simulink model "Target_Control_System"  (R2021b)
settings: Solver=FixedStepDiscrete  StartTime=0.0  StopTime=5  RelTol=1e-3
PreLoadFcn:
  | RTWConfigurationCB('preloadfcn', bdroot);
PostLoadFcn:
  | load('configuration/data_struct.mat');
  | load('configuration/fluxMaps_propMotor.mat');
  | load('configuration/parameterInit_PROP.mat');
  | load('configuration/parameterInit_PUMP.mat');
  | load('configuration/parameterInit_PITCH.mat');
  | load('configuration/parameterInit_TILT.mat');
  | %load('configuration/base_workspace_signal_definition.mat');
  | %load('resolvedatastores_to_baseworkspace_for_faster_simulation.mat');
model workspace (MAT data in the model file):
  SIMULATION_OPTIONS : Simulink.Parameter (value not decoded)
  TARGET_CODE_GEN : Simulink.Parameter (value not decoded)
  TCS_SAMPLE_FREQ_HZ : Simulink.Parameter (value not decoded)
symbols that are objects in the model workspace (value not decoded): TARGET_CODE_GEN, TCS_SAMPLE_FREQ_HZ
undefined symbols (not defined in the file): A_DQ_REF_LPF_INIT__PITCH, A_DQ_REF_LPF_INIT__PROP, A_DQ_REF_LPF_INIT__PUMP, A_DQ_REF_LPF_INIT__TILT, A_OBSERVER_CONFIDENCE_INIT__PITCH, A_OBSERVER_CONFIDENCE_INIT__PROP, A_OBSERVER_CONFIDENCE_INIT__PUMP, A_OBSERVER_CONFIDENCE_INIT__TILT, ACTUATOR_MAX_ANGLE_TRIP__PITCH, ACTUATOR_MIN_ANGLE_TRIP__PITCH, ACTUATOR_POS_SENSOR_INV_DIRECTION__PITCH, ACTUATOR_POS_SENSOR_INV_DIRECTION__TILT, ACTUATOR_POS_SENSOR_OFFSET__PITCH, ACTUATOR_POS_SENSOR_OFFSET__TILT, ADC_scaler1_baseaddr_TILT, ADC_SCALER_FLOAT_TO_FIXPOINT_EXPANSION, ANGLE_ELEC_FROM_SENSOR_OFFSET_INIT__PITCH, ANGLE_ELEC_FROM_SENSOR_OFFSET_INIT__PROP, ANGLE_ELEC_FROM_SENSOR_OFFSET_INIT__PUMP, ANGLE_ELEC_FROM_SENSOR_OFFSET_INIT__TILT, AUTO_CLEAR_FAULTS_ENABLED__PITCH, AUTO_CLEAR_FAULTS_ENABLED__PROP, AUTO_CLEAR_FAULTS_ENABLED__PUMP, AUTO_CLEAR_FAULTS_ENABLED__TILT, AUTO_CLEAR_FAULTS_WAIT_TICKS__PITCH, AUTO_CLEAR_FAULTS_WAIT_TICKS__PROP, AUTO_CLEAR_FAULTS_WAIT_TICKS__PUMP, AUTO_CLEAR_FAULTS_WAIT_TICKS__TILT, AUTO_I_ZERO_IDLE_TICKS__PITCH, AUTO_I_ZERO_IDLE_TICKS__PROP, AUTO_I_ZERO_IDLE_TICKS__PUMP, AUTO_I_ZERO_IDLE_TICKS__TILT, AUTO_I_ZERO_OFFSET_IDC_THRESHOLD__PITCH, AUTO_I_ZERO_OFFSET_IDC_THRESHOLD__PROP, AUTO_I_ZERO_OFFSET_IDC_THRESHOLD__PUMP, AUTO_I_ZERO_OFFSET_IDC_THRESHOLD__TILT, AUTO_I_ZERO_OFFSET_IPH_THRESHOLD__PITCH, AUTO_I_ZERO_OFFSET_IPH_THRESHOLD__PROP, AUTO_I_ZERO_OFFSET_IPH_THRESHOLD__PUMP, AUTO_I_ZERO_OFFSET_IPH_THRESHOLD__TILT, AUTO_SENSORLESS_SWITCHOVER_DISABLE_OMEGA, AUTO_SENSORLESS_SWITCHOVER_ENABLE_OMEGA, AUTO_SENSORLESS_SWITCHOVER_MIN_CONFIDENCE, AUXILIARY_PROTECTION_UNIT_BASEADDR__TILT, blanking_max_error_omega_INIT_PITCH, blanking_max_error_omega_INIT_TILT, blanking_max_error_position_INIT_PITCH, blanking_max_error_position_INIT_TILT, BRUTE_START_I_Q_REF_RAMP_SPEED__PITCH, BRUTE_START_I_Q_REF_RAMP_SPEED__PROP, BRUTE_START_I_Q_REF_RAMP_SPEED__PUMP, BRUTE_START_I_Q_REF_RAMP_SPEED__TILT, CONTROL_LOOP_DT_INIT__PITCH, CONTROL_LOOP_DT_INIT__PROP, CONTROL_LOOP_DT_INIT__PUMP, CONTROL_LOOP_DT_INIT__TILT, CORRECTION_FILTER_SCALE__PITCH, CORRECTION_FILTER_SCALE__PROP, CORRECTION_FILTER_SCALE__PUMP, CORRECTION_FILTER_SCALE__TILT ... (+458)
libraries: simulink x178, Reusables_Lib x24
(part 36 of 47)

== system Target_Control_System/Target_Control_System/Simulation Controls/Simulation Data Store Initialization/setupPwm()/setPwmFrequencyApplication()_pitch/setPwmFrequency()_pitch/softwareIirFilterInitialize()1 ==
  fFreq3db : Inport
  fFreqSample : Inport  Port=2
  Constant : Constant  OutDataTypeStr=single  SampleTime=-1
  Constant1 : Constant  Value=0  OutDataTypeStr=single  SampleTime=-1
  Data Store Write : DataStoreWrite  DataStoreName=oPitch  DataStoreElements=oPitch.oMot_.oState_.oFilterDataForSpeedControlIqRef_.afConstantsA_.h0  IndexOptions=Index vector (dialog)  Indices=1  OutputSizes=1
  Data Store Write1 : DataStoreWrite  DataStoreName=oPitch  DataStoreElements=oPitch.oMot_.oState_.oFilterDataForSpeedControlIqRef_.afConstantsA_.h1  IndexOptions=Index vector (dialog)  Indices=1  OutputSizes=1
  Data Store Write10 : DataStoreWrite  DataStoreName=oPitch  DataStoreElements=oPitch.oMot_.oState_.oFilterDataForSpeedControlIqRef_.fFilterOutput_  IndexOptions=Index vector (dialog)  Indices=1  OutputSizes=1
  Data Store Write2 : DataStoreWrite  DataStoreName=oPitch  DataStoreElements=oPitch.oMot_.oState_.oFilterDataForSpeedControlIqRef_.afConstantsA_.h2  IndexOptions=Index vector (dialog)  Indices=1  OutputSizes=1
  Data Store Write3 : DataStoreWrite  DataStoreName=oPitch  DataStoreElements=oPitch.oMot_.oState_.oFilterDataForSpeedControlIqRef_.afConstantsB_.h2  IndexOptions=Index vector (dialog)  Indices=1  OutputSizes=1
  Data Store Write4 : DataStoreWrite  DataStoreName=oPitch  DataStoreElements=oPitch.oMot_.oState_.oFilterDataForSpeedControlIqRef_.afConstantsB_.h1  IndexOptions=Index vector (dialog)  Indices=1  OutputSizes=1
  Data Store Write5 : DataStoreWrite  DataStoreName=oPitch  DataStoreElements=oPitch.oMot_.oState_.oFilterDataForSpeedControlIqRef_.afConstantsB_.h0  IndexOptions=Index vector (dialog)  Indices=1  OutputSizes=1
  Data Store Write6 : DataStoreWrite  DataStoreName=oPitch  DataStoreElements=oPitch.oMot_.oState_.oFilterDataForSpeedControlIqRef_.afPreviousInputs_.h0  IndexOptions=Index vector (dialog)  Indices=1  OutputSizes=1
  Data Store Write7 : DataStoreWrite  DataStoreName=oPitch  DataStoreElements=oPitch.oMot_.oState_.oFilterDataForSpeedControlIqRef_.afPreviousInputs_.h1  IndexOptions=Index vector (dialog)  Indices=1  OutputSizes=1
  Data Store Write8 : DataStoreWrite  DataStoreName=oPitch  DataStoreElements=oPitch.oMot_.oState_.oFilterDataForSpeedControlIqRef_.afPreviousOutputs_.h0  IndexOptions=Index vector (dialog)  Indices=1  OutputSizes=1
  Data Store Write9 : DataStoreWrite  DataStoreName=oPitch  DataStoreElements=oPitch.oMot_.oState_.oFilterDataForSpeedControlIqRef_.afPreviousOutputs_.h1  IndexOptions=Index vector (dialog)  Indices=1  OutputSizes=1
  Data Type Conversion{1..5} (5 alike) : DataTypeConversion  OutDataTypeStr=single
  Demux : Demux  Outputs=6
  Divide : Product  Inputs=*/  OutDataTypeStr=single
  computeCoefficientsButter() : Subsystem
  fActualFrequencyHz : Outport
  wires:
  Data Type Conversion5/1 -> Data Store Write2/1
  Data Type Conversion4/1 -> Data Store Write1/1
  Data Type Conversion3/1 -> Data Store Write3/1
  Data Type Conversion2/1 -> Data Store Write4/1
  Data Type Conversion1/1 -> Data Store Write5/1
  fFreqSample/1 -> computeCoefficientsButter()/2(dSampleFrequencyHz)
  Constant1/1 -> Data Store Write6/1, Data Store Write7/1, Data Store Write9/1, Data Store Write10/1, Data Store Write8/1
  Demux/1 -> Data Type Conversion1/1
  Demux/2 -> Data Type Conversion2/1
  Constant/1 -> Divide/1
  Divide/1 -> Data Store Write/1
  Demux/4 -> Divide/2
  Demux/3 -> Data Type Conversion3/1
  Demux/5 -> Data Type Conversion4/1
  Demux/6 -> Data Type Conversion5/1
  computeCoefficientsButter()/1(dpOutArray) -> Demux/1
  fFreq3db/1 -> computeCoefficientsButter()/1(fCutoffFrequencyHz)
  computeCoefficientsButter()/2(fFreq3db) -> fActualFrequencyHz/1

== system Target_Control_System/Target_Control_System/Simulation Controls/Simulation Data Store Initialization/setupPwm()/setPwmFrequencyApplication()_pitch/setPwmFrequency()_pitch/updateObserver()_pitch ==
  oIsr_.oParam_.fControlLoopDt_ : Inport
  fObserverLoopFilterBandwidthHz_ : Inport  Port=2
  Constant : Constant  Value=15*2*pi  OutDataTypeStr=single
  Constant1 : Constant  Value=8*2*pi  OutDataTypeStr=single
  Constant2 : Constant  Value=2*pi  OutDataTypeStr=single
  Constant3 : Constant  Value=500  OutDataTypeStr=single
  Constant4 : Constant  Value=20  OutDataTypeStr=single
  Constant5 : Constant  Value=100*2*pi  OutDataTypeStr=single
  Constant6 : Constant  Value=4*2*pi  OutDataTypeStr=single
  Constant7 : Constant  Value=0.0625  OutDataTypeStr=single
  Data Store Write : DataStoreWrite  DataStoreName=oPitch  DataStoreElements=oPitch.oIsr_.oParam_.fALpf4hpfDcBlocking_  IndexOptions=Index vector (dialog)  Indices=1  OutputSizes=1
  Data Store Write1 : DataStoreWrite  DataStoreName=oPitch  DataStoreElements=oPitch.oIsr_.oParam_.fAFluxMagnitude_  IndexOptions=Index vector (dialog)  Indices=1  OutputSizes=1
  Data Store Write2 : DataStoreWrite  DataStoreName=oPitch  DataStoreElements=oPitch.oIsr_.oParam_.fALoopfilter2_  IndexOptions=Index vector (dialog)  Indices=1  OutputSizes=1
  Data Store Write3 : DataStoreWrite  DataStoreName=oPitch  DataStoreElements=oPitch.oMot_.oParam_.fObserverLoopFilterBandwidthHz_  IndexOptions=Index vector (dialog)  Indices=1  OutputSizes=1
  Data Store Write4 : DataStoreWrite  DataStoreName=oPitch  DataStoreElements=oPitch.oIsr_.oParam_.fAOmegaFilter2_  IndexOptions=Index vector (dialog)  Indices=1  OutputSizes=1
  Data Store Write5 : DataStoreWrite  DataStoreName=oPitch  DataStoreElements=oPitch.oMot_.oParam_.fAOmegaXfilter2_  IndexOptions=Index vector (dialog)  Indices=1  OutputSizes=1
  Data Store Write6 : DataStoreWrite  DataStoreName=oPitch  DataStoreElements=oPitch.oIsr_.oParam_.oPiDataPll2_.oParameter_.fKp_  IndexOptions=Index vector (dialog)  Indices=1  OutputSizes=1
  Divide{,1,3..4} (4 alike) : Product  Inputs=**
  Divide2 : Product  Inputs=***
  Divide5 : Product  Inputs=*/
  GreaterThan : RelationalOperator  Operator=<  OutDataTypeStr=boolean  RndMeth=Simplest
  Saturation{,1..4} (5 alike) : Saturate  UpperLimit=1.0  LowerLimit=1e-6
  Switch : Switch  Criteria=u2 > Threshold
  wires:
  Divide5/1 -> Data Store Write6/1
  Constant7/1 -> Divide5/1
  Saturation4/1 -> Data Store Write5/1
  oIsr_.oParam_.fControlLoopDt_/1 -> Divide/1, Divide1/1, Divide3/1, Divide2/2, Divide5/2, Divide4/1
  Divide4/1 -> Saturation4/1
  Constant6/1 -> Divide4/2
  Saturation3/1 -> Data Store Write4/1
  Divide3/1 -> Saturation3/1
  Constant5/1 -> Divide3/2
  Switch/1 -> Data Store Write3/1, Divide2/1
  Constant3/1 -> Switch/1
  GreaterThan/1 -> Switch/2
  Constant4/1 -> GreaterThan/2
  fObserverLoopFilterBandwidthHz_/1 -> Switch/3, GreaterThan/1
  Divide2/1 -> Saturation2/1
  Saturation2/1 -> Data Store Write2/1
  Constant2/1 -> Divide2/3
  Divide1/1 -> Saturation1/1
  Saturation1/1 -> Data Store Write1/1
  Constant1/1 -> Divide1/2
  Saturation/1 -> Data Store Write/1
  Divide/1 -> Saturation/1
  Constant/1 -> Divide/2

== system Target_Control_System/Target_Control_System/Simulation Controls/Simulation Data Store Initialization/setupPwm()/setPwmFrequencyApplication()_pitch/setPwmFrequency()_pitch/updateServoObserver()_pitch ==
  oIsr_.oParam_.fControlLoopDt_ : Inport  OutDataTypeStr=double
  fOmegaEDifferentiatorBandwidthHz_ : Inport  Port=2
  Constant : Constant  OutDataTypeStr=single
  Data Store Write : DataStoreWrite  DataStoreName=oPitch  DataStoreElements=oPitch.oMot_.oState_.oPosSensor_.fOmegaEDifferentiatorBandwidthHz_  IndexOptions=Index vector (dialog)  Indices=1  OutputSizes=1
  Divide : Product  Inputs=*/  OutDataTypeStr=single
  softwareIirFilterInitialize() : Subsystem  TreatAsAtomicUnit=on
  wires:
  fOmegaEDifferentiatorBandwidthHz_/1 -> softwareIirFilterInitialize()/1(fFreq3db)
  Divide/1 -> softwareIirFilterInitialize()/2(fFreqSample)
  oIsr_.oParam_.fControlLoopDt_/1 -> Divide/2
  softwareIirFilterInitialize()/1(fActualFrequencyHz) -> Data Store Write/1
  Constant/1 -> Divide/1

== system Target_Control_System/Target_Control_System/Simulation Controls/Simulation Data Store Initialization/updateServoObserver(&oTilt)/updateServoObserver()/softwareIirFilterInitialize()/computeCoefficientsButter() ==
  fCutoffFrequencyHz : Inport  OutDataTypeStr=single
  dSampleFrequencyHz : Inport  Port=2  OutDataTypeStr=single
  Add : Sum  Inputs=+++  OutDataTypeStr=double
  Add1 : Sum  Inputs=-+
  Add2 : Sum  Inputs=+-+  OutDataTypeStr=double
  Constant : Constant  Value=0.0008  OutDataTypeStr=single
  Constant1 : Constant  Value=0.45  OutDataTypeStr=single
  Constant{5,7,9..10} (4 alike) : Constant
  Constant2 : Constant  Value=pi  OutDataTypeStr=double
  Constant3 : Constant  OutDataTypeStr=double
  Constant4 : Constant  Value=sqrt(2)  OutDataTypeStr=double
  Constant6 : Constant  OutDataTypeStr=double
  Constant8 : Constant  Value=2
  Data Type Conversion : DataTypeConversion  OutDataTypeStr=double
  Divide : Product  Inputs=**  OutDataTypeStr=single
  Divide1 : Product  Inputs=**  OutDataTypeStr=single
  Divide{3,5..6,8,10..11} (6 alike) : Product  Inputs=**  OutDataTypeStr=double
  Divide2 : Product  Inputs=*/  OutDataTypeStr=double
  Divide4 : Product  Inputs=*/  OutDataTypeStr=double
  Divide7 : Product  Inputs=*/  OutDataTypeStr=double
  Divide9 : Product  Inputs=***  OutDataTypeStr=double
  Gain : Gain  Gain=2  OutDataTypeStr=double
  Gain1 : Gain  Gain=-1  OutDataTypeStr=double
  Gain2 : Gain  Gain=-1  OutDataTypeStr=double
  Gain3 : Gain  Gain=-1  OutDataTypeStr=double
  Mux : Mux  Inputs=6
  Saturation Dynamic : simulink/Discontinuities/Saturation Dynamic  OutMin=[]  OutMax=[]  OutDataTypeStr=Inherit: Same as second input  OutDataType=fixdt(1, 16)  OutScaling=2^-10  DoSatur=off
  Tan : Trigonometry  Operator=tan
  dpOutArray : Outport
  fFreq3db : Outport  Port=2
  wires:
  Data Type Conversion/1 -> Divide2/1
  Constant10/1 -> Mux/4
  [dA2] -> Gain3/1
  Gain3/1 -> Mux/6
  [dA1] -> Gain2/1
  Gain2/1 -> Mux/5
  [dB2] -> Mux/3
  [dB1] -> Mux/2
  [dB0] -> Mux/1
  Divide11/1 -> [dA2]
  Gain1/1 -> Divide11/2
  Add2/1 -> Gain1/1
  Constant9/1 -> Add2/3
  Divide10/1 -> Add2/2
  [kdQ] -> Divide10/2
  Constant7/1 -> Add1/1
  Divide8/1 -> Add1/2, Add2/1
  Divide9/1 -> [dA1]
  Constant8/1 -> Divide9/3
  Add1/1 -> Divide9/2
  [kdIta] -> Divide8/1, Divide8/2, Divide10/1
  Gain/1 -> [dB1]
  Divide7/1 -> [dB0], Gain/1, [dB2], Divide9/1, Divide11/1
  Add/1 -> Divide7/2
  Constant6/1 -> Divide7/1
  Constant5/1 -> Add/3
  Divide5/1 -> Add/2
  Divide6/1 -> Add/1
  [kdQ] -> Divide5/2
  [kdIta] -> Divide5/1, Divide6/1, Divide6/2
  Mux/1 -> dpOutArray/1
  Constant4/1 -> [kdQ]
  Divide4/1 -> [kdIta]
  Constant3/1 -> Divide4/1
  Tan/1 -> Divide4/2
  Divide3/1 -> Tan/1
  Constant2/1 -> Divide3/2
  Divide2/1 -> Divide3/1  "dFf"
  Constant/1 -> Divide/2
  Saturation Dynamic/1 -> fFreq3db/1, Data Type Conversion/1  "fCutoffFrequencyHz"
  Divide1/1 -> Saturation Dynamic/1
  dSampleFrequencyHz/1 -> Divide1/2, Divide2/2, Divide/1
  Constant1/1 -> Divide1/1
  Divide/1 -> Saturation Dynamic/3
  fCutoffFrequencyHz/1 -> Saturation Dynamic/2

== system Target_Control_System/Target_Control_System/Simulation Controls/Simulation Data Store Initialization/updateServoObserver()/updateServoObserver()_pitch/softwareIirFilterInitialize()/computeCoefficientsButter() ==
  fCutoffFrequencyHz : Inport  OutDataTypeStr=single
  dSampleFrequencyHz : Inport  Port=2  OutDataTypeStr=single
  Add : Sum  Inputs=+++  OutDataTypeStr=double
  Add1 : Sum  Inputs=-+
  Add2 : Sum  Inputs=+-+  OutDataTypeStr=double
  Constant : Constant  Value=0.0008  OutDataTypeStr=single  SampleTime=-1
  Constant1 : Constant  Value=0.45  OutDataTypeStr=single  SampleTime=-1
  Constant{5,7,9..10} (4 alike) : Constant  SampleTime=-1
  Constant2 : Constant  Value=pi  OutDataTypeStr=double  SampleTime=-1
  Constant3 : Constant  OutDataTypeStr=double  SampleTime=-1
  Constant4 : Constant  Value=sqrt(2)  OutDataTypeStr=double  SampleTime=-1
  Constant6 : Constant  OutDataTypeStr=double  SampleTime=-1
  Constant8 : Constant  Value=2  SampleTime=-1
  Data Type Conversion : DataTypeConversion  OutDataTypeStr=double
  Divide : Product  Inputs=**  OutDataTypeStr=single
  Divide1 : Product  Inputs=**  OutDataTypeStr=single
  Divide{3,5..6,8,10..11} (6 alike) : Product  Inputs=**  OutDataTypeStr=double
  Divide2 : Product  Inputs=*/  OutDataTypeStr=double
  Divide4 : Product  Inputs=*/  OutDataTypeStr=double
  Divide7 : Product  Inputs=*/  OutDataTypeStr=double
  Divide9 : Product  Inputs=***  OutDataTypeStr=double
  Gain : Gain  Gain=2  OutDataTypeStr=double
  Gain1 : Gain  Gain=-1  OutDataTypeStr=double
  Gain2 : Gain  Gain=-1  OutDataTypeStr=double
  Gain3 : Gain  Gain=-1  OutDataTypeStr=double
  Mux : Mux  Inputs=6
  Saturation Dynamic : simulink/Discontinuities/Saturation Dynamic  OutMin=[]  OutMax=[]  OutDataTypeStr=Inherit: Same as second input  OutDataType=fixdt(1, 16)  OutScaling=2^-10  DoSatur=off
  Tan : Trigonometry  Operator=tan
  dpOutArray : Outport
  fFreq3db : Outport  Port=2
  wires:
  Data Type Conversion/1 -> Divide2/1
  Constant10/1 -> Mux/4
  [dA2] -> Gain3/1
  Gain3/1 -> Mux/6
  [dA1] -> Gain2/1
  Gain2/1 -> Mux/5
  [dB2] -> Mux/3
  [dB1] -> Mux/2
  [dB0] -> Mux/1
  Divide11/1 -> [dA2]
  Gain1/1 -> Divide11/2
  Add2/1 -> Gain1/1
  Constant9/1 -> Add2/3
  Divide10/1 -> Add2/2
  [kdQ] -> Divide10/2
  Constant7/1 -> Add1/1
  Divide8/1 -> Add1/2, Add2/1
  Divide9/1 -> [dA1]
  Constant8/1 -> Divide9/3
  Add1/1 -> Divide9/2
  [kdIta] -> Divide8/1, Divide8/2, Divide10/1
  Gain/1 -> [dB1]
  Divide7/1 -> [dB0], Gain/1, [dB2], Divide9/1, Divide11/1
  Add/1 -> Divide7/2
  Constant6/1 -> Divide7/1
  Constant5/1 -> Add/3
  Divide5/1 -> Add/2
  Divide6/1 -> Add/1
  [kdQ] -> Divide5/2
  [kdIta] -> Divide5/1, Divide6/1, Divide6/2
  Mux/1 -> dpOutArray/1
  Constant4/1 -> [kdQ]
  Divide4/1 -> [kdIta]
  Constant3/1 -> Divide4/1
  Tan/1 -> Divide4/2
  Divide3/1 -> Tan/1
  Constant2/1 -> Divide3/2
  Divide2/1 -> Divide3/1  "dFf"
  Constant/1 -> Divide/2
  Saturation Dynamic/1 -> fFreq3db/1, Data Type Conversion/1  "fCutoffFrequencyHz"
  Divide1/1 -> Saturation Dynamic/1
  dSampleFrequencyHz/1 -> Divide1/2, Divide2/2, Divide/1
  Constant1/1 -> Divide1/1
  Divide/1 -> Saturation Dynamic/3
  fCutoffFrequencyHz/1 -> Saturation Dynamic/2

== system Target_Control_System/Target_Control_System/MainLoop/pitchMotor_mainLoop/Decimation gate for 10 Hz Pitch/Function-Call Subsystem/Dynamic_current_limiting_pitch/Enabled Subsystem/Enabled Subsystem ==
  Enable : EnablePort
  Constant2 : Constant  Value=0  OutDataTypeStr=uint32  SampleTime=-1
  Constant4 : Constant  Value=0  OutDataTypeStr=uint32  SampleTime=-1
  Data Store Write5 : DataStoreWrite  DataStoreName=oPitch  DataStoreElements=oPitch.oMot_.oOut_.uiEnableGateDrive_  IndexOptions=Index vector (dialog)  Indices=1  OutputSizes=1
  Data Store Write6 : DataStoreWrite  DataStoreName=oPitch  DataStoreElements=oPitch.oMot_.oOut_.uiCurrentControllerActive_  IndexOptions=Index vector (dialog)  Indices=1  OutputSizes=1
  wires:
  Constant2/1 -> Data Store Write5/1
  Constant4/1 -> Data Store Write6/1

== system Target_Control_System/Target_Control_System/MainLoop/pitchMotor_mainLoop/Decimation gate for 200 Hz Pitch/Function-Call Subsystem/Forced current injection for broken input sensors/Enabled Subsystem/Pure_0rpm_holding_mode ==
  Enable : EnablePort
  Constant : Constant  Value=0  OutDataTypeStr=single  SampleTime=-1
  Data Store Write : DataStoreWrite  DataStoreName=oPitch  DataStoreElements=oPitch.oMot_.oState_.oRampDataOmegaERef_.fSetpoint_  IndexOptions=Index vector (dialog)  Indices=1  OutputSizes=1
  Data Store Write1 : DataStoreWrite  DataStoreName=oPitch  DataStoreElements=oPitch.oMot_.oState_.oRampDataOmegaERef_.fRampOut_  IndexOptions=Index vector (dialog)  Indices=1  OutputSizes=1
  wires:
  Constant/1 -> Data Store Write/1, Data Store Write1/1

== system Target_Control_System/Target_Control_System/MainLoop/pitchMotor_mainLoop/Decimation gate for 200 Hz Pitch/Function-Call Subsystem/Forced current injection for broken input sensors/Enabled Subsystem/Rudimentary_forced_angle_position_control ==
  note: // (fErrorReduction_ assumed to be gte 0)
  note: // Limit maximum speed
  note: // Reduce top speed 33-fold
  Enable : EnablePort
  Abs1 : Abs
  Add2 : Sum  Inputs=+-
  Add3 : Sum  Inputs=+-
  Data Store Read : DataStoreRead  DataStoreName=oPitch  DataStoreElements=oPitch.oMot_.oState_.oRampDataPos_.fRampOut_  IndexOptions=Index vector (dialog)  Indices=1  OutputSizes=1
  Data Store Read1 : DataStoreRead  DataStoreName=oPitch  DataStoreElements=oPitch.oMot_.oState_.oPosSensor_.fActuatorAngleFromSensor_  IndexOptions=Index vector (dialog)  Indices=1  OutputSizes=1
  Data Store Read2 : DataStoreRead  DataStoreName=oPitch  DataStoreElements=oPitch.oMot_.oState_.oPosSensor_.oPidDataPosCtrl_.oParameter_.fErrorReduction_  IndexOptions=Index vector (dialog)  Indices=1  OutputSizes=1
  Data Store Read3 : DataStoreRead  DataStoreName=oPitch  DataStoreElements=oPitch.oMot_.oState_.oPosSensor_.oPidDataPosCtrl_.oParameter_.fKp_  IndexOptions=Index vector (dialog)  Indices=1  OutputSizes=1
  Data Store Read4 : DataStoreRead  DataStoreName=oPitch  DataStoreElements=oPitch.oMot_.oState_.oPosSensor_.oPidDataPosCtrl_.oParameter_.fOutMax_  IndexOptions=Index vector (dialog)  Indices=1  OutputSizes=1
  Data Store Read5 : DataStoreRead  DataStoreName=oPitch  DataStoreElements=oPitch.oMot_.oState_.oPosSensor_.oPidDataPosCtrl_.oParameter_.fOutMin_  IndexOptions=Index vector (dialog)  Indices=1  OutputSizes=1
  Data Store Write : DataStoreWrite  DataStoreName=oPitch  DataStoreElements=oPitch.oMot_.oState_.oRampDataOmegaERef_.fSetpoint_  IndexOptions=Index vector (dialog)  Indices=1  OutputSizes=1
  Divide2 : Product  Inputs=**
  Divide3 : Product  Inputs=**
  Gain2 : Gain  Gain=0.03  OutDataTypeStr=single
  Gain3 : Gain  Gain=0.03  OutDataTypeStr=single
  Max1 : MinMax  Function=max  Inputs=2
  Min1 : MinMax  Inputs=2
  Saturation1 : Saturate  UpperLimit=inf  LowerLimit=0
  Sign1 : Signum
  wires:
  Max1/1 -> Data Store Write/1  "fOmegaRef"
  Gain3/1 -> Max1/2
  Min1/1 -> Max1/1
  Gain2/1 -> Min1/2
  Data Store Read5/1 -> Gain3/1
  Data Store Read4/1 -> Gain2/1
  Divide3/1 -> Min1/1  "fOmegaRef"
  Data Store Read3/1 -> Divide3/2
  Divide2/1 -> Divide3/1  "fPositionError"
  Sign1/1 -> Divide2/1
  Saturation1/1 -> Divide2/2
  Add3/1 -> Saturation1/1  "fTemp"
  Data Store Read2/1 -> Add3/2
  Abs1/1 -> Add3/1
  Add2/1 -> Abs1/1, Sign1/1  "fPositionError"
  Data Store Read/1 -> Add2/1
  Data Store Read1/1 -> Add2/2

== system Target_Control_System/Target_Control_System/MainLoop/pitchMotor_mainLoop/Decimation gate for 200 Hz Pitch/Function-Call Subsystem/Idle controller/Not forced angle/piControllerStep_Idle_Controller(&oPitch) ==
  fActual : Inport
  fTarget : Inport  Port=2
  fKp : Inport  Port=3
  fKi : Inport  Port=4
  fScale : Inport  Port=5
  fLoopDt : Inport  Port=6
  fIntMax : Inport  Port=7
  fOutMax : Inport  Port=8
  fIntMin : Inport  Port=9
  fOutMin : Inport  Port=10
  fState : Inport  Port=11
  Add : Sum  Inputs=|++
  Mux : Mux  Inputs=3
  Mux1 : Mux  Inputs=3
  Product : Product
  Saturation Dynamic : simulink/Discontinuities/Saturation Dynamic  OutMin=[]  OutMax=[]  OutDataTypeStr=Inherit: Same as second input  OutDataType=fixdt(1, 16)  OutScaling=2^-10  DoSatur=off
  Saturation Dynamic1 : simulink/Discontinuities/Saturation Dynamic  OutMin=[]  OutMax=[]  OutDataTypeStr=Inherit: Same as second input  OutDataType=fixdt(1, 16)  OutScaling=2^-10  DoSatur=off
  Scope3 : Scope  NumInputPorts=6
  Sum1 : Sum  Inputs=++|
  Sum22 : Sum  Inputs=-+|
  Unit Delay2 : UnitDelay  SampleTime=-1  HasFrameUpgradeWarning=on
  fError * fKi_ * fScale : Fcn  Expr=u(1)*u(2)*u(3)
  fError * fKp_ * fScale1 : Fcn  Expr=u(1)*u(2)*u(3)
  fOutput : Outport
  *fpState : Outport  Port=2
  wires:
  fLoopDt/1 -> Product/2
  fOutMax/1 -> Saturation Dynamic1/1
  fOutMin/1 -> Saturation Dynamic1/3
  fIntMin/1 -> Saturation Dynamic/3
  fIntMax/1 -> Saturation Dynamic/1
  Unit Delay2/1 -> Scope3/5, *fpState/1, Sum1/2
  Add/1 -> Saturation Dynamic/2
  fState/1 -> Add/2
  Product/1 -> Add/1
  Mux1/1 -> fError * fKp_ * fScale1/1
  fKi/1 -> Mux/2
  fScale/1 -> Mux/1, Mux1/3
  fKp/1 -> Mux1/2
  Mux/1 -> fError * fKi_ * fScale/1
  Saturation Dynamic1/1 -> fOutput/1, Scope3/6
  Sum1/1 -> Saturation Dynamic1/2  "fError"
  fError * fKp_ * fScale1/1 -> Sum1/1, Scope3/4
  Saturation Dynamic/1 -> Unit Delay2/1  "*fpState"
  fActual/1 -> Sum22/1, Scope3/2
  fTarget/1 -> Sum22/2, Scope3/1
  fError * fKi_ * fScale/1 -> Product/1
  Sum22/1 -> Scope3/3, Mux/3, Mux1/1  "fError"

== system Target_Control_System/Target_Control_System/MainLoop/pitchMotor_mainLoop/Decimation gate for 200 Hz Pitch/Function-Call Subsystem/Position control checks/Position control mode/Check AD2S1210 ==
  function : TriggerPort  TriggerType=function-call  VariantControl=Variant
  Data Store Read : DataStoreRead  DataStoreName=oPitch  DataStoreElements=oPitch.oMot_.oState_.oPosSensor_.eInputPositionSensorType_  IndexOptions=Index vector (dialog)  Indices=1  OutputSizes=1
  Enabled Subsystem : Subsystem  TreatAsAtomicUnit=on
  Enumerated Constant : simulink/Sources/Enumerated Constant  OutDataTypeStr=Enum: EPositionSensor_t  Value=EPositionSensor_t.eResolver  SampleTime=-1
  Equal : RelationalOperator  Operator===  OutDataTypeStr=boolean  RndMeth=Simplest
  wires:
  Equal/1 -> Enabled Subsystem/Enable
  Data Store Read/1 -> Equal/1
  Enumerated Constant/1 -> Equal/2

== system Target_Control_System/Target_Control_System/MainLoop/pitchMotor_mainLoop/Decimation gate for 200 Hz Pitch/Function-Call Subsystem/Position control checks/Position control mode/Check fighting controllers ==
  note: Check fighting controllers
      | (For dual inverter independent position control)
      | MvdG: Possibly remove again, because it is not actually in use? QAZ
  note: (ab)use the threshold setting as on-off switch too.
  function : TriggerPort  TriggerType=function-call  VariantControl=Variant
  Constant : Constant  Value=0  OutDataTypeStr=int32  SampleTime=-1
  Data Store Read : DataStoreRead  DataStoreName=oPitch  DataStoreElements=oPitch.oMot_.oState_.oPosSensor_.fFightingCurrentMagnitude_  IndexOptions=Index vector (dialog)  Indices=1  OutputSizes=1
  Enabled Subsystem : Subsystem  TreatAsAtomicUnit=on
  GreaterThan : RelationalOperator  Operator=>  OutDataTypeStr=boolean  RndMeth=Simplest
  wires:
  Constant/1 -> GreaterThan/2
  GreaterThan/1 -> Enabled Subsystem/Enable
  Data Store Read/1 -> GreaterThan/1

== system Target_Control_System/Target_Control_System/MainLoop/pitchMotor_mainLoop/Decimation gate for 200 Hz Pitch/Function-Call Subsystem/Position control checks/Position control mode/Check for position halted ==
  function : TriggerPort  TriggerType=function-call  VariantControl=Variant
  Chart1 : Stateflow chart  TreatAsAtomicUnit=on

== system Target_Control_System/Target_Control_System/MainLoop/pitchMotor_mainLoop/Decimation gate for 200 Hz Pitch/Function-Call Subsystem/Position control checks/Position control mode/checkSensorLimits(&oPitch) ==
  note: In the emergency 'ePassiveHolding' mode, iPosControlEnabled_ is false, so this will not trip
  function : TriggerPort  TriggerType=function-call  VariantControl=Variant
  Check broken sensor : Subsystem  TreatAsAtomicUnit=on
  Check delta input-output : Subsystem  TreatAsAtomicUnit=on
  Check for stuck sensor : Subsystem  TreatAsAtomicUnit=on
  Check limits : Subsystem  TreatAsAtomicUnit=on
  Function-Call Generator : simulink/Ports & Subsystems/Function-Call Generator  sample_time=-1  numberOfIterations=1  DisallowWideOutput=off
  Function-Call Split{1..3,10} (4 alike) : FunctionCallSplit  NumOutputPorts=2
  Read sensor flags : Subsystem  TreatAsAtomicUnit=on
  wires:
  Function-Call Split2/2 -> Function-Call Split3/1
  Function-Call Split10/1 -> Read sensor flags/Trigger
  Function-Call Split1/1 -> Check limits/Trigger
  Function-Call Split3/2 -> Check for stuck sensor/Trigger
  Function-Call Split1/2 -> Function-Call Split2/1
  Function-Call Split2/1 -> Check broken sensor/Trigger
  Function-Call Generator/1 -> Function-Call Split10/1
  Function-Call Split3/1 -> Check delta input-output/Trigger
  Function-Call Split10/2 -> Function-Call Split1/1

== system Target_Control_System/Target_Control_System/MainLoop/pitchMotor_mainLoop/Decimation gate for 5000 Hz Pitch/motorTaskProcessExternalSetpoints(&oPitch)/set_target/Id_target/Subsystem ==
  Input : Inport
  Enable : EnablePort
  Data Store Read1 : DataStoreRead  DataStoreName=oPitch  DataStoreElements=oPitch.oMot_.oParam_.fISetpointMax_  IndexOptions=Index vector (dialog)  Indices=1  OutputSizes=1
  Data Store Read74 : DataStoreRead  DataStoreName=oPitch  DataStoreElements=oPitch.oMot_.oParam_.fISetpointMax_  IndexOptions=Index vector (dialog)  Indices=1  OutputSizes=1
  Data Store Write1 : DataStoreWrite  DataStoreName=oPitch  DataStoreElements=oPitch.oMot_.oState_.fIdExternalSetpoint_  IndexOptions=Index vector (dialog)  Indices=1  OutputSizes=1
  Gain2 : Gain  Gain=-1
  Saturation Dynamic : simulink/Discontinuities/Saturation Dynamic  OutMin=[]  OutMax=[]  OutDataTypeStr=Inherit: Same as second input  OutDataType=fixdt(1, 16)  OutScaling=2^-10  DoSatur=off
  wires:
  Data Store Read1/1 -> Gain2/1
  Data Store Read74/1 -> Saturation Dynamic/1
  Gain2/1 -> Saturation Dynamic/3
  Input/1 -> Saturation Dynamic/2
  Saturation Dynamic/1 -> Data Store Write1/1

== system Target_Control_System/Target_Control_System/MainLoop/pitchMotor_mainLoop/Decimation gate for 5000 Hz Pitch/motorTaskProcessExternalSetpoints(&oPitch)/set_target/Iq_target/Subsystem ==
  Enable : EnablePort
  Data Store Read1 : DataStoreRead  DataStoreName=oPitch  DataStoreElements=oPitch.oMot_.oParam_.fIqSetpointMax_  IndexOptions=Index vector (dialog)  Indices=1  OutputSizes=1
  Data Store Read68 : DataStoreRead  DataStoreName=oPitch  DataStoreElements=oPitch.oMot_.oIn_.fIqSetpoint_  IndexOptions=Index vector (dialog)  Indices=1  OutputSizes=1
  Data Store Read74 : DataStoreRead  DataStoreName=oPitch  DataStoreElements=oPitch.oMot_.oParam_.fIqSetpointMax_  IndexOptions=Index vector (dialog)  Indices=1  OutputSizes=1
  Data Store Read81 : DataStoreRead  DataStoreName=oPitch  DataStoreElements=oPitch.oMot_.oParam_.fDynILimIntegratorLeakageFactor_  IndexOptions=Index vector (dialog)  Indices=1  OutputSizes=1
  Data Store Write19 : DataStoreWrite  DataStoreName=oPitch  DataStoreElements=oPitch.oMot_.oState_.fIqRefBeforeRamp_  IndexOptions=Index vector (dialog)  Indices=1  OutputSizes=1
  Dynamic Current Limiting Prop : Subsystem  TreatAsAtomicUnit=on
  Gain2 : Gain  Gain=-1
  Saturation Dynamic : simulink/Discontinuities/Saturation Dynamic  OutMin=[]  OutMax=[]  OutDataTypeStr=Inherit: Same as second input  OutDataType=fixdt(1, 16)  OutScaling=2^-10  DoSatur=off
  Switch4 : Switch  Criteria=u2 > Threshold
  wires:
  Dynamic Current Limiting Prop/1(fIqRefBeforeRamp_) -> Switch4/1
  Switch4/1 -> Data Store Write19/1
  Data Store Read81/1 -> Dynamic Current Limiting Prop/Enable, Switch4/2
  Gain2/1 -> Saturation Dynamic/3
  Data Store Read74/1 -> Saturation Dynamic/1
  Data Store Read68/1 -> Saturation Dynamic/2
  Data Store Read1/1 -> Gain2/1
  Saturation Dynamic/1 -> Switch4/3

== system Target_Control_System/Target_Control_System/MainLoop/pitchMotor_mainLoop/Decimation gate for 5000 Hz Pitch/motorTaskProcessExternalSetpoints(&oPitch)/set_target/position_target/Subsystem ==
  Enable : EnablePort
  Current Limiting Prop : Subsystem  TreatAsAtomicUnit=on
  Data Store Read2 : DataStoreRead  DataStoreName=oPitch  DataStoreElements=oPitch.oMot_.oIn_.fPosSetpoint_  IndexOptions=Index vector (dialog)  Indices=1  OutputSizes=1
  Data Store Read85 : DataStoreRead  DataStoreName=oPitch  DataStoreElements=oPitch.oMot_.oState_.uiDriveState_  IndexOptions=Index vector (dialog)  Indices=1  OutputSizes=1
  Data Store Write1 : DataStoreWrite  DataStoreName=oPitch  DataStoreElements=oPitch.oMot_.oState_.oRampDataPos_.fSetpoint_  IndexOptions=Index vector (dialog)  Indices=1  OutputSizes=1
  Equal13 : RelationalOperator  Operator=~=  OutDataTypeStr=boolean  RndMeth=Simplest
  const17 : Constant  Value=228  OutDataTypeStr=uint32  SampleTime=-1
  wires:
  Equal13/1 -> Current Limiting Prop/Enable
  const17/1 -> Equal13/1
  Data Store Read85/1 -> Equal13/2
  Data Store Read2/1 -> Data Store Write1/1, Current Limiting Prop/1(oRampDataPos_.fSetpoint_)

== system Target_Control_System/Target_Control_System/MainLoop/pitchMotor_mainLoop/Decimation gate for 5000 Hz Pitch/motorTaskProcessExternalSetpoints(&oPitch)/set_target/speed_target/Subsystem ==
  Enable : EnablePort
  Data Store Read1 : DataStoreRead  DataStoreName=oPitch  DataStoreElements=oPitch.oMot_.oParam_.fPolePairs_  IndexOptions=Index vector (dialog)  Indices=1  OutputSizes=1
  Data Store Read2 : DataStoreRead  DataStoreName=oPitch  DataStoreElements=oPitch.oMot_.oIn_.fRpmSetpoint_  IndexOptions=Index vector (dialog)  Indices=1  OutputSizes=1
  Data Store Read3 : DataStoreRead  DataStoreName=oPitch  DataStoreElements=oPitch.oMot_.oParam_.fOmegaESetpointMax_  IndexOptions=Index vector (dialog)  Indices=1  OutputSizes=1
  Data Store Read74 : DataStoreRead  DataStoreName=oPitch  DataStoreElements=oPitch.oMot_.oParam_.fOmegaESetpointMax_  IndexOptions=Index vector (dialog)  Indices=1  OutputSizes=1
  Data Store Write1 : DataStoreWrite  DataStoreName=oPitch  DataStoreElements=oPitch.oMot_.oState_.oRampDataOmegaERef_.fSetpoint_  IndexOptions=Index vector (dialog)  Indices=1  OutputSizes=1
  Gain : Gain  Gain=-1
  Product : Product  Inputs=3
  Saturation Dynamic : simulink/Discontinuities/Saturation Dynamic  OutMin=[]  OutMax=[]  OutDataTypeStr=Inherit: Same as second input  OutDataType=fixdt(1, 16)  OutScaling=2^-10  DoSatur=off
  const1 : Constant  Value=0.10471975512  OutDataTypeStr=single  SampleTime=-1
  wires:
  Saturation Dynamic/1 -> Data Store Write1/1
  Product/1 -> Saturation Dynamic/2
  Data Store Read3/1 -> Gain/1
  Gain/1 -> Saturation Dynamic/3
  Data Store Read74/1 -> Saturation Dynamic/1
  const1/1 -> Product/2
  Data Store Read1/1 -> Product/3
  Data Store Read2/1 -> Product/1

== system Target_Control_System/Target_Control_System/MainLoop/pitchMotor_mainLoop/mainTask_pitch/motorTaskMainFastStep()/Automatic switching to sensorless - Pitch/Automatic switching to sensorless/Switch to sensored  ==
  note: // Presently enabled, do we need to disable?
  fObserverConfidence : Inport
  Action Port : ActionPort
  Abs1 : Abs
  Data Store Read28 : DataStoreRead  DataStoreName=oPitch  DataStoreElements=oPitch.oMot_.oIn_.fOmegaEObserverRaw2_  IndexOptions=Index vector (dialog)  Indices=1  OutputSizes=1
  Data Store Read29 : DataStoreRead  DataStoreName=oPitch  DataStoreElements=oPitch.oMot_.oParam_.fAutoSensorlessSwitchoverDisableOmega_  IndexOptions=Index vector (dialog)  Indices=1  OutputSizes=1
  Data Store Read42 : DataStoreRead  DataStoreName=oPitch  DataStoreElements=oPitch.oMot_.oParam_.fAutoSensorlessSwitchoverMinConfidence_  IndexOptions=Index vector (dialog)  Indices=1  OutputSizes=1
  Less Than : RelationalOperator  Operator=<  OutDataTypeStr=boolean  RndMeth=Simplest
  Less Than1 : RelationalOperator  Operator=<  OutDataTypeStr=boolean  RndMeth=Simplest
  OR : Logic  Operator=OR  AllPortsSameDT=off  OutDataTypeStr=boolean
  Switch to sensored : Subsystem  TreatAsAtomicUnit=on
  wires:
  OR/1 -> Switch to sensored/Enable
  fObserverConfidence/1 -> Less Than1/1
  Data Store Read29/1 -> Less Than/2
  Data Store Read42/1 -> Less Than1/2
  Abs1/1 -> Less Than/1
  Less Than/1 -> OR/1
  Data Store Read28/1 -> Abs1/1
  Less Than1/1 -> OR/2

== system Target_Control_System/Target_Control_System/MainLoop/pitchMotor_mainLoop/mainTask_pitch/motorTaskMainFastStep()/Automatic switching to sensorless - Pitch/Automatic switching to sensorless/Switch to sensorless? ==
  fObserverConfidence : Inport
  Action Port : ActionPort
  Abs1 : Abs
  Data Store Read28 : DataStoreRead  DataStoreName=oPitch  DataStoreElements=oPitch.oMot_.oIn_.fOmegaEObserverRaw2_  IndexOptions=Index vector (dialog)  Indices=1  OutputSizes=1
  Data Store Read29 : DataStoreRead  DataStoreName=oPitch  DataStoreElements=oPitch.oMot_.oParam_.fAutoSensorlessSwitchoverEnableOmega_  IndexOptions=Index vector (dialog)  Indices=1  OutputSizes=1
  Data Store Read42 : DataStoreRead  DataStoreName=oPitch  DataStoreElements=oPitch.oMot_.oParam_.fAutoSensorlessSwitchoverMinConfidence_  IndexOptions=Index vector (dialog)  Indices=1  OutputSizes=1
  Less Than : RelationalOperator  Operator=>  OutDataTypeStr=boolean  RndMeth=Simplest
  Less Than1 : RelationalOperator  Operator=>  OutDataTypeStr=boolean  RndMeth=Simplest
  OR : Logic  AllPortsSameDT=off  OutDataTypeStr=boolean
  Switch to sensorless : Subsystem  TreatAsAtomicUnit=on
  wires:
  Less Than/1 -> OR/1
  Data Store Read42/1 -> Less Than1/2
  Less Than1/1 -> OR/2
  fObserverConfidence/1 -> Less Than1/1
  Data Store Read29/1 -> Less Than/2
  Data Store Read28/1 -> Abs1/1
  Abs1/1 -> Less Than/1
  OR/1 -> Switch to sensorless/Enable

== system Target_Control_System/Target_Control_System/MainLoop/pitchMotor_mainLoop/mainTask_pitch/motorTaskMainFastStep()/Control Loops - Pitch/Position Controller Pitch/Connect PosController to CurrentController ==
  fPMultiplier : Inport
  fIMultiplier : Inport  Port=2
  DMultiplier : Inport  Port=3
  fITerm : Inport  Port=4
  fDTerm : Inport  Port=5
  fPTerm : Inport  Port=6
  Add : Sum  Inputs=+++
  Divide : Product  Inputs=**
  Divide1 : Product  Inputs=**
  Divide2 : Product  Inputs=**
  fIqRefFromSpeedController : Outport
  wires:
  Add/1 -> fIqRefFromSpeedController/1
  Divide2/1 -> Add/3
  Divide/1 -> Add/1
  Divide1/1 -> Add/2
  fDTerm/1 -> Divide2/1
  DMultiplier/1 -> Divide2/2
  fITerm/1 -> Divide1/1
  fIMultiplier/1 -> Divide1/2
  fPMultiplier/1 -> Divide/2
  fPTerm/1 -> Divide/1

== system Target_Control_System/Target_Control_System/MainLoop/pitchMotor_mainLoop/mainTask_pitch/motorTaskMainFastStep()/Control Loops - Pitch/Position Controller Pitch/pid2ControllerStep(oPidDataPosCtrl)_pitch ==
  fActual : Inport
  fTarget : Inport  Port=2
  fErrorReduction : Inport  Port=3
  fLargeErrorThresholdPositive : Inport  Port=4
  fLargeErrorThresholdNegative : Inport  Port=5
  fBlankingMaxError : Inport  Port=6
  fKi : Inport  Port=7
  ipInhibitTarget : Inport  Port=8
  fLoopDt : Inport  Port=9
  fIntMax : Inport  Port=10
  fIntMin : Inport  Port=11
  fIntegratorLeakFactor : Inport  Port=12
  fKd : Inport  Port=13
  fActualDt : Inport  Port=14
  fDMax : Inport  Port=15
  fDMin : Inport  Port=16
  fKp : Inport  Port=17
  fOutMax : Inport  Port=18
  fOutMin : Inport  Port=19
  fpState : Inport  Port=20
  Abs : Abs
  Abs1 : Abs
  Add : Sum  Inputs=|++
  Add1 : Sum
  Constant : Constant  Value=0  OutDataTypeStr=single
  Constant3 : Constant  Value=0  OutDataTypeStr=single
  Constant4 : Constant  Value=0  OutDataTypeStr=single
  Constant5 : Constant  OutDataTypeStr=single
  Constant6 : Constant  OutDataTypeStr=int32
  Constant7 : Constant  Value=-1  OutDataTypeStr=int32
  Constant8 : Constant  Value=0  OutDataTypeStr=int32
  Divide : Product  Inputs=**
  Divide1 : Product  Inputs=**
  GreaterThan2 : RelationalOperator  OutDataTypeStr=boolean  RndMeth=Simplest
  GreaterThan3 : RelationalOperator  Operator=>  OutDataTypeStr=boolean  RndMeth=Simplest
  GreaterThan4 : RelationalOperator  Operator=>  OutDataTypeStr=boolean  RndMeth=Simplest
  GreaterThan5 : RelationalOperator  Operator=<  OutDataTypeStr=boolean  RndMeth=Simplest
  GreaterThan6 : RelationalOperator  Operator=<  OutDataTypeStr=boolean  RndMeth=Simplest
  GreaterThan7 : RelationalOperator  Operator=>  OutDataTypeStr=boolean  RndMeth=Simplest
  GreaterThan8 : RelationalOperator  Operator=<  OutDataTypeStr=boolean  RndMeth=Simplest
  OR1 : Logic  AllPortsSameDT=off  OutDataTypeStr=boolean
  OR2 : Logic  AllPortsSameDT=off  OutDataTypeStr=boolean
  OR3 : Logic  Operator=OR  AllPortsSameDT=off  OutDataTypeStr=boolean
  Product{,1..4} (5 alike) : Product
  Saturation : Saturate  UpperLimit=inf  LowerLimit=0
  Saturation Dynamic : simulink/Discontinuities/Saturation Dynamic  OutMin=[]  OutMax=[]  OutDataTypeStr=Inherit: Same as second input  OutDataType=fixdt(1, 16)  OutScaling=2^-10  DoSatur=off
  Saturation Dynamic1 : simulink/Discontinuities/Saturation Dynamic  OutMin=[]  OutMax=[]  OutDataTypeStr=Inherit: Same as second input  OutDataType=fixdt(1, 16)  OutScaling=2^-10  DoSatur=off
  Saturation Dynamic2 : simulink/Discontinuities/Saturation Dynamic  OutMin=[]  OutMax=[]  OutDataTypeStr=Inherit: Same as second input  OutDataType=fixdt(1, 16)  OutScaling=2^-10  DoSatur=off
  Sign : Signum
  Sum : Sum  Inputs=|++
  Sum2 : Sum  Inputs=-+|
  Sum22 : Sum  Inputs=-+|
  Sum4 : Sum  Inputs=+-|
  Switch{1..4} (4 alike) : Switch  Criteria=u2 > Threshold
  Unit Delay2 : UnitDelay  SampleTime=-1  HasFrameUpgradeWarning=on
  iLargeErrorPresent : Outport
  fITerm : Outport  Port=2
  fDTerm : Outport  Port=3
  fPTerm : Outport  Port=4
  fOutput : Outport  Port=5
  *fpState : Outport  Port=6
  wires:
  Switch3/1 -> iLargeErrorPresent/1
  Constant6/1 -> Switch4/1
  GreaterThan8/1 -> Switch3/2
  GreaterThan7/1 -> Switch4/2
  Switch4/1 -> Switch3/3
  Constant8/1 -> Switch4/3
  Constant7/1 -> Switch3/1
  Sum/1 -> Saturation Dynamic1/2
  Add1/1 -> Sum/2
  Product4/1 -> fPTerm/1, Sum/1
  fKp/1 -> Product4/1
  Saturation Dynamic2/1 -> fDTerm/1, Add1/1  "fDTerm"
  fDMax/1 -> Saturation Dynamic2/1
  fDMin/1 -> Saturation Dynamic2/3
  Product3/1 -> Saturation Dynamic2/2  "fDTerm"
  fActualDt/1 -> Product3/2
  fKd/1 -> Product3/1
  Unit Delay2/1 -> Product2/1  "*fpState"
  Product2/1 -> fITerm/1, *fpState/1, Add1/2  "*fpState"
  Sum4/1 -> Product2/2
  Constant5/1 -> Sum4/1
  Product1/1 -> Sum4/2
  fIntegratorLeakFactor/1 -> Product1/2
  Saturation Dynamic/1 -> Unit Delay2/1
  Add/1 -> Saturation Dynamic/2  "fpState"
  Switch2/1 -> Product/1  "fErrorForIntegrator"
  Constant4/1 -> Switch2/1
  OR3/1 -> Switch2/2
  OR2/1 -> OR3/2
  OR1/1 -> OR3/1
  GreaterThan6/1 -> OR2/2
  GreaterThan5/1 -> OR2/1
  GreaterThan3/1 -> OR1/2
  GreaterThan4/1 -> OR1/1
  Divide1/1 -> GreaterThan4/1, Switch2/3, GreaterThan5/1  "fErrorForIntegrator"
  Constant3/1 -> GreaterThan3/2, GreaterThan4/2, GreaterThan5/2, GreaterThan6/2
  ipInhibitTarget/1 -> GreaterThan6/1, GreaterThan3/1
  fKi/1 -> Divide1/2
  Switch1/1 -> Divide1/1  "fErrorForIntegrator"
  Constant/1 -> Switch1/3
  GreaterThan2/1 -> Switch1/2
  fBlankingMaxError/1 -> GreaterThan2/2
  Abs1/1 -> GreaterThan2/1
  fLargeErrorThresholdNegative/1 -> GreaterThan8/2
  fLargeErrorThresholdPositive/1 -> GreaterThan7/2
  Divide/1 -> Product4/2, GreaterThan8/1, Abs1/1, Switch1/1, GreaterThan7/1  "fError"
  Sign/1 -> Divide/2
  Saturation/1 -> Divide/1
  Sum2/1 -> Saturation/1  "fTemp"
  fErrorReduction/1 -> Sum2/1
  Abs/1 -> Sum2/2
  fActual/1 -> Sum22/1
  fOutMax/1 -> Saturation Dynamic1/1
  fpState/1 -> Add/2
  Saturation Dynamic1/1 -> fOutput/1
  fTarget/1 -> Sum22/2
  Product/1 -> Add/1
  Sum22/1 -> Abs/1, Sign/1  "fError"
  fOutMin/1 -> Saturation Dynamic1/3
  fIntMax/1 -> Saturation Dynamic/1
  fLoopDt/1 -> Product/2, Product1/1
  fIntMin/1 -> Saturation Dynamic/3

== system Target_Control_System/Target_Control_System/MainLoop/pitchMotor_mainLoop/mainTask_pitch/motorTaskMainFastStep()/Control Loops - Pitch/Speed Controller Pitch/Enabled Subsystem ==
  oRampDataOmegaERef_.fRampOut : Inport
  Enable : EnablePort
  Constant1 : Constant  OutDataTypeStr=single  SampleTime=-1
  Data Store Read10 : DataStoreRead  DataStoreName=oPitch  DataStoreElements=oPitch.oMot_.oParam_.oPid2DataRpmCtrl_.oParameter_.fLargeErrorThresholdNegative_  IndexOptions=Index vector (dialog)  Indices=1  OutputSizes=1
  Data Store Read12 : DataStoreRead  DataStoreName=oPitch  DataStoreElements=oPitch.oMot_.oParam_.oPid2DataRpmCtrl_.oParameter_.fBlankingMaxError_  IndexOptions=Index vector (dialog)  Indices=1  OutputSizes=1
  Data Store Read14 : DataStoreRead  DataStoreName=oPitch  DataStoreElements=oPitch.oMot_.oParam_.oPid2DataRpmCtrl_.oParameter_.fKi_  IndexOptions=Index vector (dialog)  Indices=1  OutputSizes=1
  Data Store Read15 : DataStoreRead  DataStoreName=oPitch  DataStoreElements=oPitch.oMot_.oParam_.oPid2DataRpmCtrl_.oParameter_.fLoopDt_  IndexOptions=Index vector (dialog)  Indices=1  OutputSizes=1
  Data Store Read16 : DataStoreRead  DataStoreName=oPitch  DataStoreElements=oPitch.oMot_.oParam_.oPid2DataRpmCtrl_.oParameter_.fIntMax_  IndexOptions=Index vector (dialog)  Indices=1  OutputSizes=1
  Data Store Read17 : DataStoreRead  DataStoreName=oPitch  DataStoreElements=oPitch.oMot_.oParam_.oPid2DataRpmCtrl_.oParameter_.fIntMin_  IndexOptions=Index vector (dialog)  Indices=1  OutputSizes=1
  Data Store Read18 : DataStoreRead  DataStoreName=oPitch  DataStoreElements=oPitch.oMot_.oParam_.oPid2DataRpmCtrl_.oParameter_.ipInhibitTarget_  IndexOptions=Index vector (dialog)  Indices=1  OutputSizes=1
  Data Store Read19 : DataStoreRead  DataStoreName=oPitch  DataStoreElements=oPitch.oMot_.oParam_.oPid2DataRpmCtrl_.oParameter_.fIntegratorLeakFactor_  IndexOptions=Index vector (dialog)  Indices=1  OutputSizes=1
  Data Store Read20 : DataStoreRead  DataStoreName=oPitch  DataStoreElements=oPitch.oMot_.oParam_.oPid2DataRpmCtrl_.oParameter_.fKd_  IndexOptions=Index vector (dialog)  Indices=1  OutputSizes=1
  Data Store Read21 : DataStoreRead  DataStoreName=oPitch  DataStoreElements=oPitch.oMot_.oParam_.oPid2DataRpmCtrl_.oParameter_.fDMax_  IndexOptions=Index vector (dialog)  Indices=1  OutputSizes=1
  Data Store Read22 : DataStoreRead  DataStoreName=oPitch  DataStoreElements=oPitch.oMot_.oParam_.oPid2DataRpmCtrl_.oParameter_.fDMin_  IndexOptions=Index vector (dialog)  Indices=1  OutputSizes=1
  Data Store Read23 : DataStoreRead  DataStoreName=oPitch  DataStoreElements=oPitch.oMot_.oParam_.oPid2DataRpmCtrl_.oParameter_.fKp_  IndexOptions=Index vector (dialog)  Indices=1  OutputSizes=1
  Data Store Read24 : DataStoreRead  DataStoreName=oPitch  DataStoreElements=oPitch.oMot_.oParam_.oPid2DataRpmCtrl_.oParameter_.fOutMin_  IndexOptions=Index vector (dialog)  Indices=1  OutputSizes=1
  Data Store Read3 : DataStoreRead  DataStoreName=oPitch  DataStoreElements=oPitch.oMot_.oParam_.oPid2DataRpmCtrl_.oParameter_.fOutMax_  IndexOptions=Index vector (dialog)  Indices=1  OutputSizes=1
  Data Store Read4 : DataStoreRead  DataStoreName=oPitch  DataStoreElements=oPitch.oMot_.oParam_.oPid2DataRpmCtrl_.fState_  IndexOptions=Index vector (dialog)  Indices=1  OutputSizes=1
  Data Store Read7 : DataStoreRead  DataStoreName=oPitch  DataStoreElements=oPitch.oMot_.oState_.oPosSensor_.fOmegaEFromSensor_  IndexOptions=Index vector (dialog)  Indices=1  OutputSizes=1
  Data Store Read8 : DataStoreRead  DataStoreName=oPitch  DataStoreElements=oPitch.oMot_.oParam_.oPid2DataRpmCtrl_.oParameter_.fErrorReduction_  IndexOptions=Index vector (dialog)  Indices=1  OutputSizes=1
  Data Store Read9 : DataStoreRead  DataStoreName=oPitch  DataStoreElements=oPitch.oMot_.oParam_.oPid2DataRpmCtrl_.oParameter_.fLargeErrorThresholdPositive_  IndexOptions=Index vector (dialog)  Indices=1  OutputSizes=1
  Data Store Write : DataStoreWrite  DataStoreName=oPitch  DataStoreElements=oPitch.oMot_.oParam_.oPid2DataRpmCtrl_.oParameter_.iLargeErrorPresent_  IndexOptions=Index vector (dialog)  Indices=1  OutputSizes=1
  Data Store Write1 : DataStoreWrite  DataStoreName=oPitch  DataStoreElements=oPitch.oMot_.oParam_.oPid2DataRpmCtrl_.oParameter_.fITerm_  IndexOptions=Index vector (dialog)  Indices=1  OutputSizes=1
  Data Store Write2 : DataStoreWrite  DataStoreName=oPitch  DataStoreElements=oPitch.oMot_.oParam_.oPid2DataRpmCtrl_.oParameter_.fDTerm_  IndexOptions=Index vector (dialog)  Indices=1  OutputSizes=1
  Data Store Write3 : DataStoreWrite  DataStoreName=oPitch  DataStoreElements=oPitch.oMot_.oParam_.oPid2DataRpmCtrl_.oParameter_.fPTerm_  IndexOptions=Index vector (dialog)  Indices=1  OutputSizes=1
  Data Store Write4 : DataStoreWrite  DataStoreName=oPitch  DataStoreElements=oPitch.oMot_.oState_.fIqRefFromSpeedController_  IndexOptions=Index vector (dialog)  Indices=1  OutputSizes=1
  Data Store Write5 : DataStoreWrite  DataStoreName=oPitch  DataStoreElements=oPitch.oMot_.oParam_.oPid2DataRpmCtrl_.fState_  IndexOptions=Index vector (dialog)  Indices=1  OutputSizes=1
  pid2ControllerStep(oPidDataRpmCtrl)_pitch : Subsystem  TreatAsAtomicUnit=on
  fIqRefFromSpeedController : Outport
  wires:
  oRampDataOmegaERef_.fRampOut/1 -> pid2ControllerStep(oPidDataRpmCtrl)_pitch/2(fTarget)
  Data Store Read15/1 -> pid2ControllerStep(oPidDataRpmCtrl)_pitch/9(fLoopDt)
  Data Store Read8/1 -> pid2ControllerStep(oPidDataRpmCtrl)_pitch/3(fErrorReduction)
  pid2ControllerStep(oPidDataRpmCtrl)_pitch/4(fPTerm) -> Data Store Write3/1
  Data Store Read9/1 -> pid2ControllerStep(oPidDataRpmCtrl)_pitch/4(fLargeErrorThresholdPositive)
  Data Store Read7/1 -> pid2ControllerStep(oPidDataRpmCtrl)_pitch/1(fActual)
  Data Store Read14/1 -> pid2ControllerStep(oPidDataRpmCtrl)_pitch/7(fKi)
  pid2ControllerStep(oPidDataRpmCtrl)_pitch/3(fDTerm) -> Data Store Write2/1
  Data Store Read17/1 -> pid2ControllerStep(oPidDataRpmCtrl)_pitch/11(fIntMin)
  pid2ControllerStep(oPidDataRpmCtrl)_pitch/6(*fpState) -> Data Store Write5/1
  Data Store Read23/1 -> pid2ControllerStep(oPidDataRpmCtrl)_pitch/17(fKp)
  pid2ControllerStep(oPidDataRpmCtrl)_pitch/5(fOutput) -> Data Store Write4/1, fIqRefFromSpeedController/1
  Data Store Read22/1 -> pid2ControllerStep(oPidDataRpmCtrl)_pitch/16(fDMin)
  Data Store Read20/1 -> pid2ControllerStep(oPidDataRpmCtrl)_pitch/13(fKd)
  Data Store Read19/1 -> pid2ControllerStep(oPidDataRpmCtrl)_pitch/12(fIntegratorLeakFactor)
  Data Store Read18/1 -> pid2ControllerStep(oPidDataRpmCtrl)_pitch/8(ipInhibitTarget)
  pid2ControllerStep(oPidDataRpmCtrl)_pitch/2(fITerm) -> Data Store Write1/1
  Data Store Read24/1 -> pid2ControllerStep(oPidDataRpmCtrl)_pitch/19(fOutMin)
  pid2ControllerStep(oPidDataRpmCtrl)_pitch/1(iLargeErrorPresent) -> Data Store Write/1
  Data Store Read3/1 -> pid2ControllerStep(oPidDataRpmCtrl)_pitch/18(fOutMax)
  Constant1/1 -> pid2ControllerStep(oPidDataRpmCtrl)_pitch/14(fActualDt)
  Data Store Read16/1 -> pid2ControllerStep(oPidDataRpmCtrl)_pitch/10(fIntMax)
  Data Store Read21/1 -> pid2ControllerStep(oPidDataRpmCtrl)_pitch/15(fDMax)
  Data Store Read4/1 -> pid2ControllerStep(oPidDataRpmCtrl)_pitch/20(fpState)
  Data Store Read12/1 -> pid2ControllerStep(oPidDataRpmCtrl)_pitch/6(fBlankingMaxError)
  Data Store Read10/1 -> pid2ControllerStep(oPidDataRpmCtrl)_pitch/5(fLargeErrorThresholdNegative)
